simulink model "velo_id_gain_tc_simu"  (R2020b)
settings: Solver=VariableStepAuto  StartTime=0.0  StopTime=10.0  RelTol=1e-3
values from neighbouring files (symbols this model uses):
  p_const = 0.7    [velo_id_gain.m]    (also in velo_id_gain_tc.m = 0.5; velo_id_tc.m = 0.5; velo_id_verify.m = 1; velo_pi_mbd.m = 1)
  r_const = 0.7    [velo_id_gain.m]    (also in velo_id_gain_tc.m = 1.3; velo_id_tc.m = 1.3; velo_id_verify.m = 0.75)
  s_time = 10    [velo_id_gain.m]    (also in velo_id_gain_tc.m; velo_id_tc.m; velo_id_verify.m; velo_pi_mbd.m = 5)
  u_ini = 1.5    [velo_id_gain_tc.m]    (also in velo_id_tc.m)
libraries: arduino_io_lib x4
settings Model: Creator=kei55  LastModifiedBy=kei55

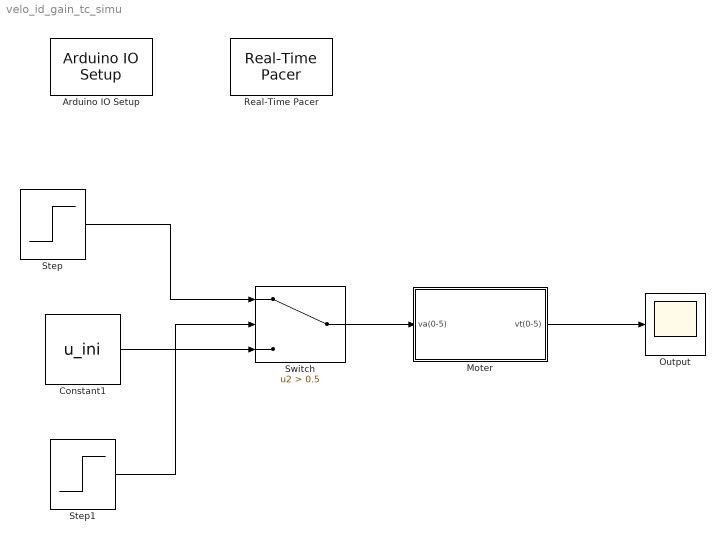
== system velo_id_gain_tc_simu ==
  Arduino IO Setup : arduino_io_lib/Arduino IO Setup  Priority=3  arduinoVar=Temporary arduino variable: Arduino1  workspaceVarName=a  comPort=COM3
  Constant1 : Constant  Value=u_ini
  Moter : Subsystem
  Output : Scope
  Real-Time Pacer : arduino_io_lib/Real-Time Pacer  simTimePerRealTime=1
  Step : Step  Time=s_time  Before=r_const  After=r_const+p_const  SampleTime=0
  Step1 : Step  Time=s_time  Before=r_const  After=r_const+p_const  SampleTime=0
  Switch : Switch  Criteria=u2 > Threshold  Threshold=0.5
  wires:
  Moter/1(vt(0-5)) -> Output/1
  Switch/1 -> Moter/1(va(0-5))
  Constant1/1 -> Switch/3
  Step/1 -> Switch/1
  Step1/1 -> Switch/2

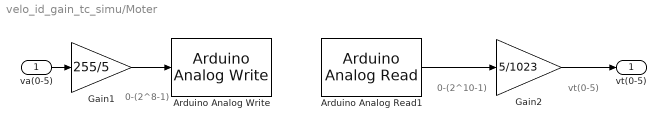
== system velo_id_gain_tc_simu/Moter ==
  note: 0-(2^8-1)
  note: 0-(2^10-1)
  note: vt(0-5)
  va(0-5) : Inport
  Arduino Analog Read1 : arduino_io_lib/Arduino Analog Read  arduinoVar=Temporary arduino variable: Arduino1  arduinoPin=0  T=1/50
  Arduino Analog Write : arduino_io_lib/Arduino Analog Write  arduinoVar=Temporary arduino variable: Arduino1  arduinoPin=3  T=1/50
  Gain1 : Gain  Gain=255/5
  Gain2 : Gain  Gain=5/1023
  vt(0-5) : Outport
  wires:
  Arduino Analog Read1/1 -> Gain2/1
  Gain1/1 -> Arduino Analog Write/1
  Gain2/1 -> vt(0-5)/1
  va(0-5)/1 -> Gain1/1
